simulink model "dpd_adapt_verify"  (R2024a)
settings: Solver=FixedStepDiscrete  StartTime=0.0  StopTime=inf  RelTol=1e-3
PreLoadFcn:
  | load rpem_dpd_coef  % variable = dpd_coef
  | filter_num=[ .25]*exp(j*pi/4);     % phase offset
  | filter_den=[1 -.75*(1+j)/sqrt(2)]; % complex denominator
  | MK=5*5;  % 5x5 DPD size
  | C_init=complex(zeros(MK,1))+.1;  % initial DPD coefficients
  | 
  | % LMS algorithm parameters
  | Mu=0.2;    % LMS gain
  | 
  | % RPEM algorithm parameters
  | L0=0.99;
  | L_init=0.95;
  | p=0.8;
  | P0=p*complex(eye(MK));
StartFcn:
  | tic
StopFcn:
  | trun=toc
  | n=1:length(dpd_coef);
  | plot(n,real(dpd_coef),n,imag(dpd_coef))
  | xlabel('index');
  | ylabel(' Real and Imaginary parts of DPD Coefficients')
  | title('DPD Coefficients');
  | legend('real','imag')
undefined symbols (not defined in the file): dfilt, dpd_coef, fdesignblkfcn, gcbh
libraries: dspstat3 x4, dspobslib x4, commrflib2 x2, ILA_CONFIGSS x1, commchan3 x1, dsparch4 x1, simulink x1, commutil2 x1, dspmathops x1
settings Model: Creator=Dick  LastModifiedBy=10938
settings SolverCC: AlgebraicLoopSolver=TrustRegion
settings DataIOCC: LimitDataPoints=on  SaveFormat=Array  SaveOutput=off  SaveTime=off  ReturnWorkspaceOutputs=off
settings OptimizationCC: BlockReduction=off  ConditionallyExecuteInputs=off  DefaultParameterBehavior=Inlined  ExpressionDepthLimit=2147483647  LifeSpan=inf  SimCompilerOptimization=on
settings DebuggingCC: AlgebraicLoopMsg=error  UnderspecifiedInitializationDetection=Classic  MergeDetectMultiDrivingBlocksExec=none  SolverPrmCheckMsg=warning  InheritedTsInSrcMsg=none  MultiTaskRateTransMsg=warning  ParameterPrecisionLossMsg=none  FcnCallInpInsideContextMsg=warning  UnconnectedLineMsg=warning  StateNameClashWarn=warning  SFUnexpectedBacktrackingDiag=warning  SFNoUnconditionalDefaultTransitionDiag=warning  SFExecutionAtInitializationDiag=none  ArithmeticOperatorsInVariantConditions=warning
settings HardwareCC: ProdBitPerPointer=32  ProdBitPerSizeT=32  ProdBitPerPtrDiffT=32  ProdLargestAtomicFloat=None  ProdIntDivRoundTo=Undefined  ProdEndianess=Unspecified  ProdWordSize=32  ProdHWDeviceType=ASIC/FPGA->ASIC/FPGA  ProdEqTarget=off
settings ModelReferenceCC: PropagateSignalLabelsOutOfModel=off
settings SFSimCC: SimCtrlC=off  SimUseLocalCustomCode=off  CustomCodeUndefinedFunction=UseInterfaceOnly
settings RTWCC: RTWUseLocalCustomCode=off  GPUComputeCapability=3.5
settings CodeAppCC: StateflowObjectComments=on
settings GRTTargetCC: TargetLangStandard=C89/C90 (ANSI)  CombineOutputUpdateFcns=off  GRTInterface=on
settings ConfigComp: CovMetricSettings=dw  CovSaveCumulativeToWorkspaceVar=on  CovSaveSingleToWorkspaceVar=on  CovExternalEMLEnable=off  CovSFcnEnable=off

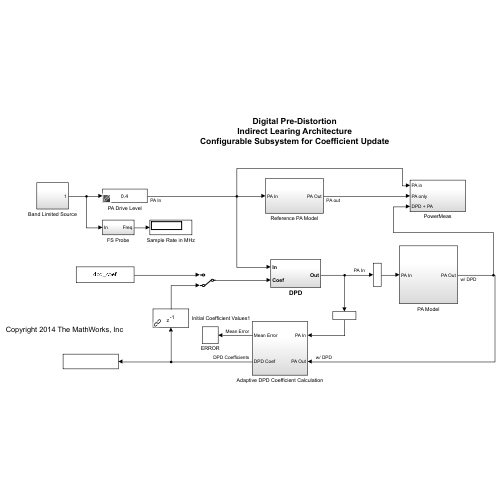
[thumbnail: Simulink's stored preview of the top-level diagram]
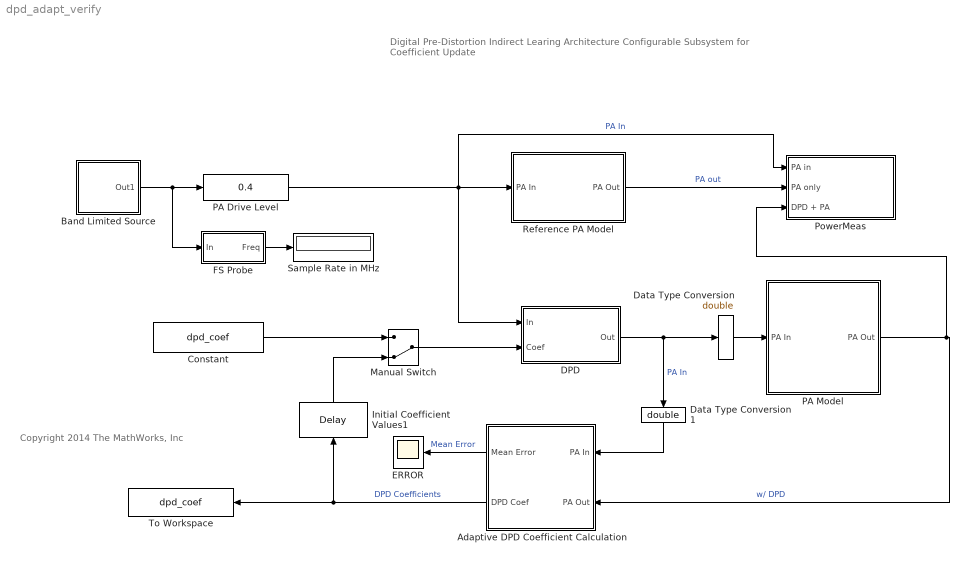
== system dpd_adapt_verify ==
  note: Copyright 2014 The MathWorks, Inc
  note: Digital Pre-Distortion
      | Indirect Learing Architecture
      | Configurable Subsystem for Coefficient Update
  Adaptive DPD Coefficient Calculation : Subsystem
  Band Limited Source : Subsystem
  Constant : Constant  Value=dpd_coef  SampleTime=1/(10e6)
  DPD : Subsystem
  Data Type Conversion : DataTypeConversion  OutDataTypeStr=double  SaturateOnIntegerOverflow=off  RndMeth=Floor
  Data Type Conversion1 : DataTypeConversion  OutDataTypeStr=double  SaturateOnIntegerOverflow=off  RndMeth=Floor
  ERROR : Scope
  FS Probe : Subsystem
  Initial Coefficient Values1 : dspobslib/Delay  dly_unit=Samples  delay=1  ic_detail=off  dif_ic_for_ch=on  dif_ic_for_dly=off  ic=C_init  reset_popup=None
  Manual Switch : ManualSwitch  CurrentSetting=0
  PA Drive Level : simulink/Math Operations/Slider Gain  gain=0.4  low=0  high=1
  PA Model : Subsystem
  PowerMeas : Subsystem  RequirementInfo={} %GIDa_e4fbdf0e_58e4_4736_b6e2_993c187d2e03
  Reference PA Model : Subsystem
  Sample Rate in MHz : Display
  To Workspace : ToWorkspace  VariableName=dpd_coef  SampleTime=-1
      settings: MaxDataPoints=1
  wires:
  Adaptive DPD Coefficient Calculation/1(Mean Error) -> ERROR/1  "Mean Error"
  FS Probe/1(Freq) -> Sample Rate in MHz/1
  PA Model/1(PA Out) -> PowerMeas/3(DPD + PA), Adaptive DPD Coefficient Calculation/2(PA Out)  "w/ DPD"
  Band Limited Source/1(Out1) -> FS Probe/1(In), PA Drive Level/1
  DPD/1(Out) -> Data Type Conversion/1, Data Type Conversion1/1  "PA In"
  Adaptive DPD Coefficient Calculation/2(DPD Coef) -> Initial Coefficient Values1/1, To Workspace/1  "DPD Coefficients"
  PA Drive Level/1 -> PowerMeas/1(PA in), Reference PA Model/1(PA In), DPD/1(In)  "PA In"
  Data Type Conversion/1 -> PA Model/1(PA In)
  Data Type Conversion1/1 -> Adaptive DPD Coefficient Calculation/1(PA In)
  Manual Switch/1 -> DPD/2(Coef)
  Initial Coefficient Values1/1 -> Manual Switch/2
  Constant/1 -> Manual Switch/1
  Reference PA Model/1(PA Out) -> PowerMeas/2(PA only)  "PA out"

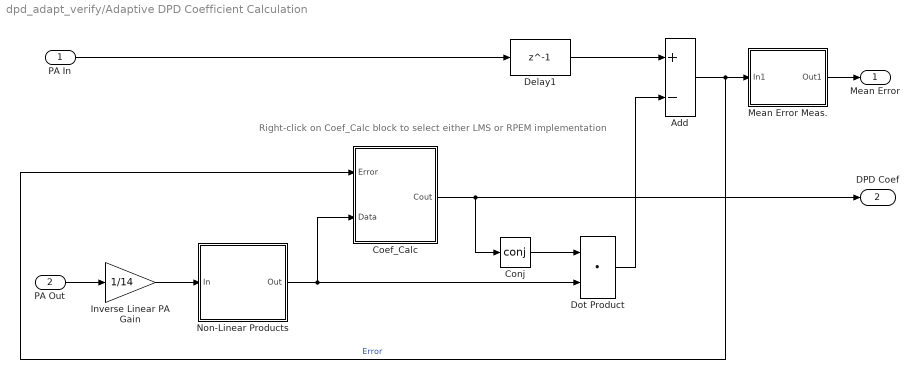
== system dpd_adapt_verify/Adaptive DPD Coefficient Calculation ==
  note: Right-click on Coef_Calc block to select either LMS or RPEM implementation
  PA In : Inport
  PA Out : Inport  Port=2
  Add : Sum  Inputs=+-
  Coef_Calc : Subsystem  BlockChoice=RPEM
      settings: AttributesFormatString=%<BlockChoice>  TemplateBlock=ILA_CONFIGSS/Coef_Calc  MemberBlocks=LMS,RPEM
  Conj : Math  Operator=conj  SignedPower=on
  Delay1 : Delay  DelayLength=1  InitialCondition=.1  UseCircularBuffer=on
  Dot Product : DotProduct  OutDataTypeStr=Inherit: Inherit via internal rule
  Inverse Linear PA Gain : Gain  Gain=1/14
  Mean Error Meas. : Subsystem
  Non-Linear Products : Subsystem
  Mean Error : Outport
  DPD Coef : Outport  Port=2
  wires:
  Add/1 -> Coef_Calc/1(Error), Mean Error Meas./1(In1)  "Error"
  Dot Product/1 -> Add/2
  Inverse Linear PA Gain/1 -> Non-Linear Products/1(In)
  Delay1/1 -> Add/1
  Non-Linear Products/1(Out) -> Coef_Calc/2(Data), Dot Product/2
  Coef_Calc/1(Cout) -> DPD Coef/1, Conj/1
  PA In/1 -> Delay1/1
  PA Out/1 -> Inverse Linear PA Gain/1
  Mean Error Meas./1(Out1) -> Mean Error/1
  Conj/1 -> Dot Product/1

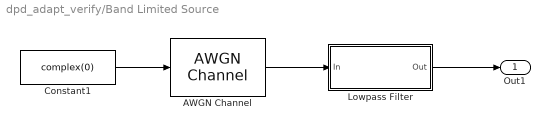
== system dpd_adapt_verify/Band Limited Source ==
  AWGN Channel : commchan3/AWGN Channel  LegacyMode=on  NoiseMethod="Signal to noise ratio  (SNR)"  noiseMode=Variance from mask  EbNo=10  EsNo=10  SNR=10  BitsPerSymbol=1  SignalPower=1  SamplesPerSymbol=1  SymbolPeriod=1  VarianceSource=Parameter  Variance=1  RandomStream=Global stream  Seed=67  SimulateUsing=Code generation
  Constant1 : Constant  Value=complex(0)  VectorParams1D=off  SampleTime=1/(10e6)
  Lowpass Filter : Subsystem  DialogController=fdesignblkfcn  InitFcn=fdesignblkfcn(gcbh, {'InitFcn'});  mask(Lowpass Filter){}
      mask help: Design a lowpass filter
      settings: CopyFcn=fdesignblkfcn(gcbh, {'CopyFcn'});
      mask Help: helpview(mapfilelocation('dsp'), 'dsplowpassfilter');
      mask Display: disp('Lowpass')
  Out1 : Outport
  wires:
  Constant1/1 -> AWGN Channel/1
  Lowpass Filter/1(Out) -> Out1/1
  AWGN Channel/1 -> Lowpass Filter/1(In)

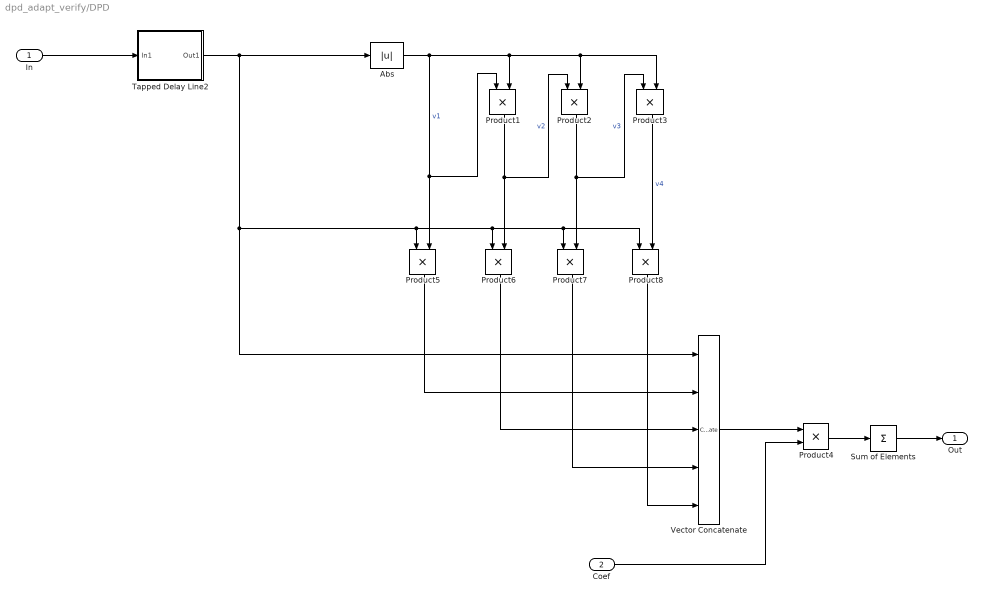
== system dpd_adapt_verify/DPD ==
  In : Inport
  Coef : Inport  Port=2
  Abs : Abs  SaturateOnIntegerOverflow=off
  Product{1..3,5..8} (7 alike) : Product  RndMeth=Zero
  Product4 : Product  OutDataTypeStr=double
  Sum of Elements : Sum  Inputs=+  OutDataTypeStr=double
  Tapped Delay Line2 : Subsystem
  Vector Concatenate : Concatenate  NumInputs=5
  Out : Outport
  wires:
  Sum of Elements/1 -> Out/1
  Coef/1 -> Product4/2
  Vector Concatenate/1 -> Product4/1
  Product4/1 -> Sum of Elements/1
  Abs/1 -> Product3/2, Product2/2, Product1/2, Product1/1, Product5/2  "v1"
  Product1/1 -> Product2/1, Product6/2  "v2"
  Product2/1 -> Product3/1, Product7/2  "v3"
  Product3/1 -> Product8/2  "v4"
  Product5/1 -> Vector Concatenate/2
  Product6/1 -> Vector Concatenate/3
  Product7/1 -> Vector Concatenate/4
  Product8/1 -> Vector Concatenate/5
  Tapped Delay Line2/1(Out1) -> Abs/1, Product8/1, Product7/1, Product6/1, Product5/1, Vector Concatenate/1
  In/1 -> Tapped Delay Line2/1(In1)

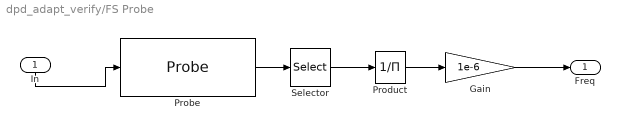
== system dpd_adapt_verify/FS Probe ==
  In : Inport
  Gain : Gain  Gain=1e-6
  Probe : Probe  ProbeWidth=off  ProbeComplexSignal=off
  Product : Product  Inputs=/
  Selector : Selector  InputPortWidth=2  IndexOptions=Index vector (dialog)  Indices=1  OutputSizes=1
  Freq : Outport
  wires:
  Selector/1 -> Product/1
  Product/1 -> Gain/1
  In/1 -> Probe/1
  Probe/1 -> Selector/1
  Gain/1 -> Freq/1

== system dpd_adapt_verify/PA Model ==
  PA In : Inport
  Asymetrical Complex Filter : dspobslib/Digital Filter  TypePopup=IIR (poles & zeros)  IIRFiltStruct=Direct form II transposed  AllPoleFiltStruct=Direct form  FIRFiltStruct=Direct form  CoeffSource=Specify via dialog  NumCoeffs="[0 filter_num]  % additional unit delay"  DenCoeffs=filter_den  BiQuadCoeffs=[1 0.3 0.4 1 0.1 0.2]  LatticeCoeffs=[0.2 0.4]  denIgnore=on  FiltPerSampPopup=One filter per frame  IC=0  ICnum=0  ICden=0  roundingMode=Floor  overflowMode=off  ScaleValues=1  scaleValueFracLength=14  stageInFracLength=15  stageOutFracLength=15  FilterSource=Specify via dialog  dfiltObjectName=dfilt.dffir([1 2 1])  InputProcessing=Columns as channels (frame based)
  Memoryless Nonlinearity : commrflib2/Memoryless Nonlinearity  Model=Saleh  LinearGainDB=0  TOI_Type=IIP3  IIP3=40  OIP3=Inf  IP1dB=Inf  OP1dB=Inf  IPsat=Inf  OPsat=Inf  Table=[ -25, 5, -1; -10, 20, -2; 0, 27, 5; 5, 28, 12 ]  MagnitudeGainDB=0  Vsat=1  MagnitudeSmooth=0.5  PhaseGainRadian=-.45  PhaseSaturation=.88  PhaseSmooth=3.43  InputScaleDB=-10  AmAmParameters=[2.1587 1.1517]  AmPmParameters=[4.0033 9.1040]  OutputScaleDB=31  ReferenceLoad=1  SimulateUsing=Code generation
  PA Out : Outport
  wires:
  Asymetrical Complex Filter/1 -> Memoryless Nonlinearity/1
  PA In/1 -> Asymetrical Complex Filter/1
  Memoryless Nonlinearity/1 -> PA Out/1

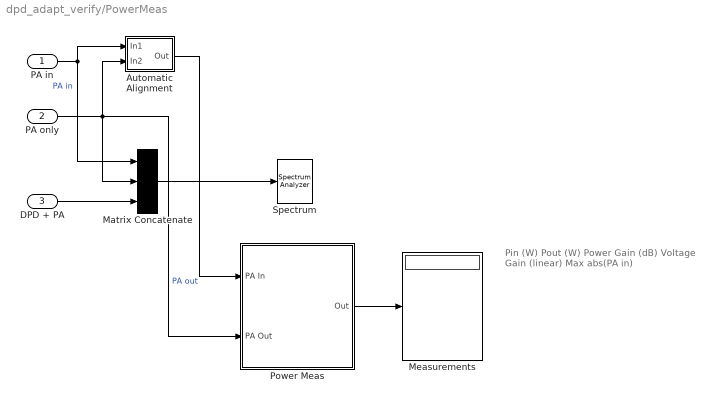
== system dpd_adapt_verify/PowerMeas ==
  note: Pin (W)
      | Pout (W)
      | Power Gain (dB)
      | Voltage Gain (linear)
      | Max abs(PA in)
  PA in : Inport
  PA only : Inport  Port=2
  DPD + PA : Inport  Port=3
  " Spectrum" : SpectrumAnalyzer  Method=Welch  AveragingMethod=Running  DefaultConfigurationName=spbscopes.SpectrumAnalyzerBlockCfg
  Automatic Alignment : Subsystem
  Matrix Concatenate : Concatenate  NumInputs=3  Mode=Multidimensional array  ConcatenateDimension=2
  Measurements : Display
  Power Meas : Subsystem
  wires:
  Matrix Concatenate/1 -> " Spectrum"/1
  PA in/1 -> Automatic Alignment/1(In1), Matrix Concatenate/1  "PA in"
  PA only/1 -> Power Meas/2(PA Out), Automatic Alignment/2(In2), Matrix Concatenate/2  "PA out"
  Automatic Alignment/1(Out) -> Power Meas/1(PA In)
  Power Meas/1(Out) -> Measurements/1
  DPD + PA/1 -> Matrix Concatenate/3

== system dpd_adapt_verify/Reference PA Model ==
  PA In : Inport
  Asymetrical Complex Filter1 : dspobslib/Digital Filter  TypePopup=IIR (poles & zeros)  IIRFiltStruct=Direct form II transposed  AllPoleFiltStruct=Direct form  FIRFiltStruct=Direct form  CoeffSource=Specify via dialog  NumCoeffs="[0 filter_num]  % additional unit delay"  DenCoeffs=filter_den  BiQuadCoeffs=[1 0.3 0.4 1 0.1 0.2]  LatticeCoeffs=[0.2 0.4]  denIgnore=on  FiltPerSampPopup=One filter per frame  IC=0  ICnum=0  ICden=0  roundingMode=Floor  overflowMode=off  ScaleValues=1  scaleValueFracLength=14  stageInFracLength=15  stageOutFracLength=15  FilterSource=Specify via dialog  dfiltObjectName=dfilt.dffir([1 2 1])  InputProcessing=Columns as channels (frame based)
  Memoryless Nonlinearity : commrflib2/Memoryless Nonlinearity  Model=Saleh  LinearGainDB=0  TOI_Type=IIP3  IIP3=40  OIP3=Inf  IP1dB=Inf  OP1dB=Inf  IPsat=Inf  OPsat=Inf  Table=[ -25, 5, -1; -10, 20, -2; 0, 27, 5; 5, 28, 12 ]  MagnitudeGainDB=0  Vsat=1  MagnitudeSmooth=0.5  PhaseGainRadian=-.45  PhaseSaturation=.88  PhaseSmooth=3.43  InputScaleDB=-10  AmAmParameters=[2.1587 1.1517]  AmPmParameters=[4.0033 9.1040]  OutputScaleDB=31  ReferenceLoad=1  SimulateUsing=Code generation
  PA Out : Outport
  wires:
  Memoryless Nonlinearity/1 -> PA Out/1
  PA In/1 -> Asymetrical Complex Filter1/1
  Asymetrical Complex Filter1/1 -> Memoryless Nonlinearity/1

== system dpd_adapt_verify/Adaptive DPD Coefficient Calculation/Coef_Calc ==
  Error : Inport
  Data : Inport  Port=2
  RPEM : ILA_CONFIGSS/RPEM
  Cout : Outport
  wires:
  Error/1 -> RPEM/1
  Data/1 -> RPEM/2
  RPEM/1 -> Cout/1

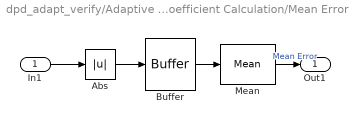
== system dpd_adapt_verify/Adaptive DPD Coefficient Calculation/Mean Error Meas. ==
  In1 : Inport
  Abs : Abs  SaturateOnIntegerOverflow=off
  Buffer : Buffer
  Mean : dspstat3/Mean  run=off  InputProcessing=Columns as channels (frame based)  reset_popup=None  directionMode=Each column  dimension=1  roiEnable=off  roiType=Rectangles  roiPortion=Entire ROI  roiOutput=Individual statistics for each ROI  roiFlag=off  roundingMode=Floor  overflowMode=off  outputDataTypeStr=Inherit: Same as accumulator  outputMin=[]  outputMax=[]  outputLastDataTypeStr=Inherit: Same as accumulator
  Out1 : Outport
  wires:
  Abs/1 -> Buffer/1
  Buffer/1 -> Mean/1
  In1/1 -> Abs/1
  Mean/1 -> Out1/1  "Mean Error"

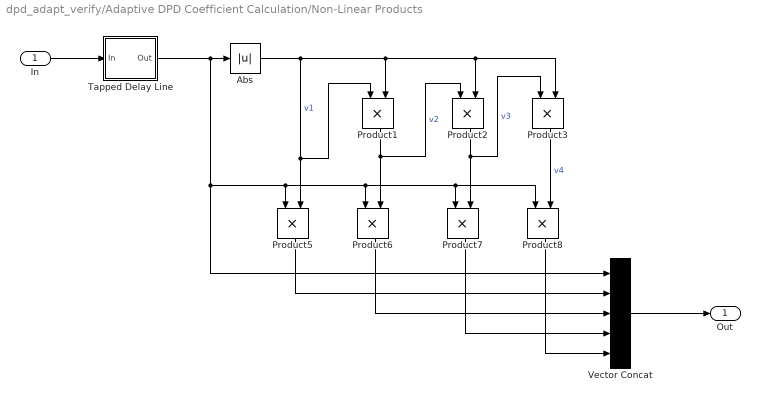
== system dpd_adapt_verify/Adaptive DPD Coefficient Calculation/Non-Linear Products ==
  In : Inport
  Abs : Abs  SaturateOnIntegerOverflow=off
  Product{1..3,5..8} (7 alike) : Product  RndMeth=Zero
  Tapped Delay Line : Subsystem
  Vector Concat : Concatenate  NumInputs=5
  Out : Outport
  wires:
  Product5/1 -> Vector Concat/2
  Product3/1 -> Product8/2  "v4"
  Product2/1 -> Product7/2, Product3/1  "v3"
  Product1/1 -> Product6/2, Product2/1  "v2"
  Abs/1 -> Product3/2, Product2/2, Product1/2, Product1/1, Product5/2  "v1"
  Vector Concat/1 -> Out/1
  Product6/1 -> Vector Concat/3
  Product8/1 -> Vector Concat/5
  Product7/1 -> Vector Concat/4
  Tapped Delay Line/1(Out) -> Abs/1, Vector Concat/1, Product5/1, Product6/1, Product7/1, Product8/1
  In/1 -> Tapped Delay Line/1(In)

== system dpd_adapt_verify/Band Limited Source/Lowpass Filter ==
  In : Inport
  Generated Filter Block : dsparch4/Biquad Filter  Tag=BlockMethodSubSystem  FilterSource=Dialog parameters  CoeffSource=Specify via dialog  FilterObject=dfilt.df2tsos([1 0.3 0.4],[1 0.1 0.2])  IIRFiltStruct=Direct form II  BiQuadCoeffs=[0.59857121639186728 0.13537231817349551 0.59857121639186728 1 -0.91924875050540011 0.79125023824409946;0.071302617967318405 0.071302617967318405 0 1 -0.72689076105008177 0;1.9999999999999993 -0.61982790413552502 2 1 -0.61172653799164256 0.97438669274901857;0.10076583159845166 0.11489786555202355 0.10076583159845166 1 -1.2555266743020157 0.62505447110737744;2 -0.34405123549902639 1.9999999999999996 1 -0.69965198413855145 0.90732338685750258]  ScaleValues=[0.17872347192286847;1;1;1;1;1.090516053438453]  IC=0  ICnum=0  ICden=0  a0Flag=Warning  optimizeScaleValues=off  ScaleValueMode=Specify via input port (g)  InputProcessing=Columns as channels (frame based)  roundingMode=Floor  overflowMode=off  scaleValueFracLength=14  denProdOutputFracLength=30  denAccumFracLength=30  secondMemoryFracLength=15
  Out : Outport
  wires:
  In/1 -> Generated Filter Block/1
  Generated Filter Block/1 -> Out/1

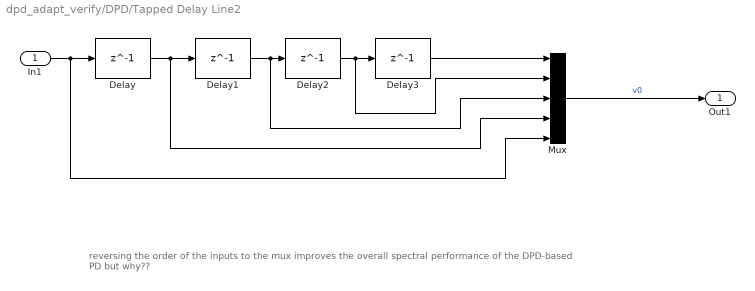
== system dpd_adapt_verify/DPD/Tapped Delay Line2 ==
  note: reversing the order of the inputs to the mux improves the overall spectral performance of the DPD-based PD but why??
  In1 : Inport
  Delay{,1..3} (4 alike) : Delay  DelayLength=1  InitialCondition=0  UseCircularBuffer=on
  Mux : Mux  Inputs=5
  Out1 : Outport
  wires:
  Delay3/1 -> Mux/1
  Mux/1 -> Out1/1  "v0"
  Delay2/1 -> Mux/2, Delay3/1
  Delay1/1 -> Mux/3, Delay2/1
  Delay/1 -> Mux/4, Delay1/1
  In1/1 -> Mux/5, Delay/1

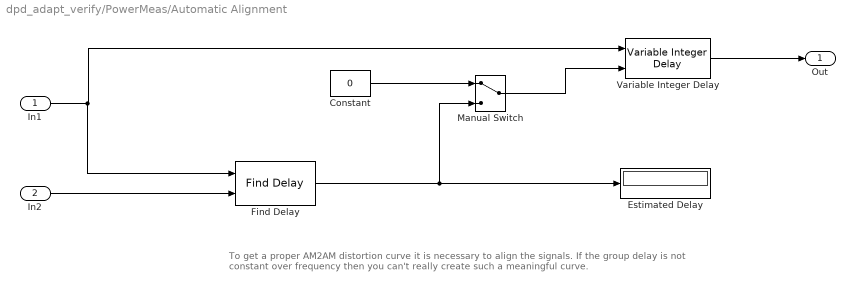
== system dpd_adapt_verify/PowerMeas/Automatic Alignment ==
  note: To get a proper AM2AM distortion curve it is necessary to align the signals. If the group delay is not constant over frequency then
      | you can't really create such a meaningful curve.
  In1 : Inport
  In2 : Inport  Port=2
  Constant : Constant  Value=0  SampleTime=1/(10e6)
  Estimated Delay : Display
  Find Delay : commutil2/Find Delay  corrLength=20  chgSigOP=off  stopUpdate=off  numConstDelay=3
  Manual Switch : ManualSwitch
  Variable Integer Delay : dspobslib/Variable Integer Delay  dmax=1024  InputProcessing=Columns as channels (frame based)  ic=0  noDFT=off
  Out : Outport
  wires:
  Find Delay/1 -> Manual Switch/2, Estimated Delay/1
  In1/1 -> Find Delay/1, Variable Integer Delay/1
  Variable Integer Delay/1 -> Out/1
  In2/1 -> Find Delay/2
  Constant/1 -> Manual Switch/1
  Manual Switch/1 -> Variable Integer Delay/2

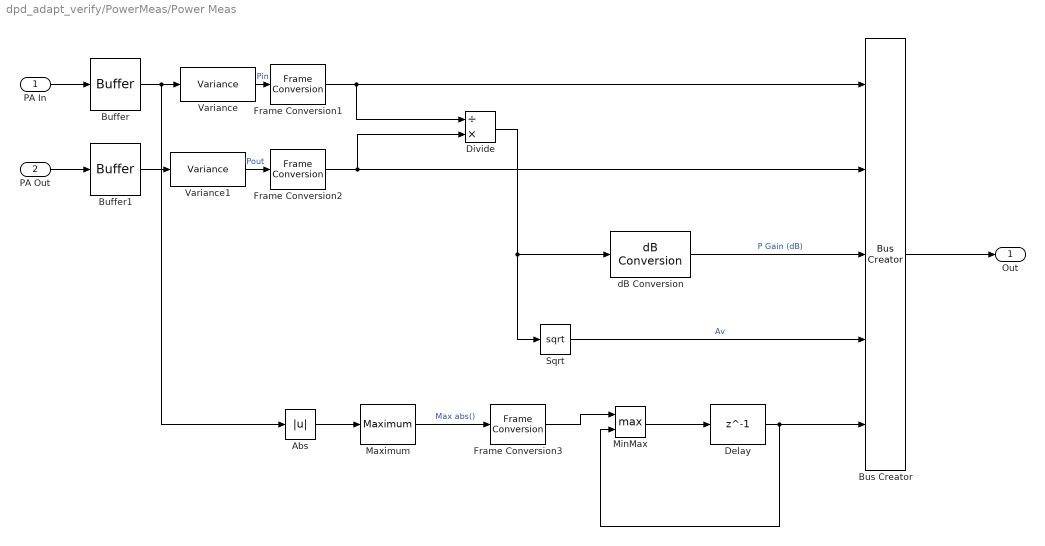
== system dpd_adapt_verify/PowerMeas/Power Meas ==
  PA In : Inport
  PA Out : Inport  Port=2
  Abs : Abs  SaturateOnIntegerOverflow=off
  Buffer : Buffer  N=1000
  Buffer1 : Buffer  N=1000
  Bus Creator : BusCreator  Inputs=5
  Delay : Delay  DelayLength=1  InitialCondition=0  InputProcessing=Columns as channels (frame based)
  Divide : Product  Inputs=/*
  Frame Conversion1 : FrameConversion  OutFrame=Sample-based
  Frame Conversion2 : FrameConversion  OutFrame=Sample-based
  Frame Conversion3 : FrameConversion  OutFrame=Sample-based
  Maximum : dspstat3/Maximum  operation=maximum  fcn=Value  indexBase=One  operateOver=Each column  Dimension=1  InputProcessing=Columns as channels (frame based)  reset=None  roiEnable=off  roiType=Rectangles  roiPortion=Entire ROI  roiOutput=Individual statistics for each ROI  roiFlag=off  roundingMode=Floor  overflowMode=off  accumDataTypeStr=Inherit: Same as product output  accumLastDataTypeStr=Inherit: Same as product output
  MinMax : MinMax  Function=max  Inputs=2
  Sqrt : Sqrt
  Variance : dspstat3/Variance  run=off  InputProcessing=Columns as channels (frame based)  reset_popup=None  directionMode=Each column  dimension=1  roiEnable=off  roiType=Rectangles  roiPortion=Entire ROI  roiOutput=Individual statistics for each ROI  roiFlag=off  roundingMode=Floor  overflowMode=off
  Variance1 : dspstat3/Variance  run=off  InputProcessing=Columns as channels (frame based)  reset_popup=None  directionMode=Each column  dimension=1  roiEnable=off  roiType=Rectangles  roiPortion=Entire ROI  roiOutput=Individual statistics for each ROI  roiFlag=off  roundingMode=Floor  overflowMode=off
  dB Conversion : dspmathops/dB Conversion  dBtype=dB  intype=Power  R=1  fuzz=off
  Out : Outport
  wires:
  Variance/1 -> Frame Conversion1/1  "Pin"
  PA In/1 -> Buffer/1
  PA Out/1 -> Buffer1/1
  Buffer1/1 -> Variance1/1
  Variance1/1 -> Frame Conversion2/1  "Pout"
  Divide/1 -> Sqrt/1, dB Conversion/1
  dB Conversion/1 -> Bus Creator/3  "P Gain (dB)"
  Sqrt/1 -> Bus Creator/4  "Av"
  Bus Creator/1 -> Out/1
  Frame Conversion1/1 -> Divide/1, Bus Creator/1
  Frame Conversion2/1 -> Divide/2, Bus Creator/2
  Abs/1 -> Maximum/1
  Maximum/1 -> Frame Conversion3/1  "Max abs()"
  Buffer/1 -> Abs/1, Variance/1
  MinMax/1 -> Delay/1
  Delay/1 -> Bus Creator/5, MinMax/2
  Frame Conversion3/1 -> MinMax/1

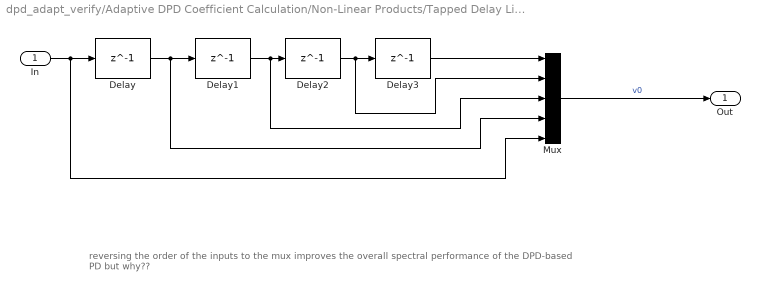
== system dpd_adapt_verify/Adaptive DPD Coefficient Calculation/Non-Linear Products/Tapped Delay Line ==
  note: reversing the order of the inputs to the mux improves the overall spectral performance of the DPD-based PD but why??
  In : Inport
  Delay{,1..3} (4 alike) : Delay  DelayLength=1  InitialCondition=0  UseCircularBuffer=on
  Mux : Mux  Inputs=5
  Out : Outport
  wires:
  In/1 -> Delay/1, Mux/5
  Delay/1 -> Delay1/1, Mux/4
  Delay1/1 -> Delay2/1, Mux/3
  Delay2/1 -> Delay3/1, Mux/2
  Mux/1 -> Out/1  "v0"
  Delay3/1 -> Mux/1
